simulink model "OCFC"  (R2023a)
settings: Solver=VariableStepAuto  StartTime=0.0  StopTime=200  RelTol=1e-3
libraries: simulink x1, slpidlib x1, SignalEditorBlockLib x1
settings Model: Creator=nineday  LastModifiedBy=nineday
settings ModelReferenceCC: EnableRefExpFcnMdlSchedulingChecks=on

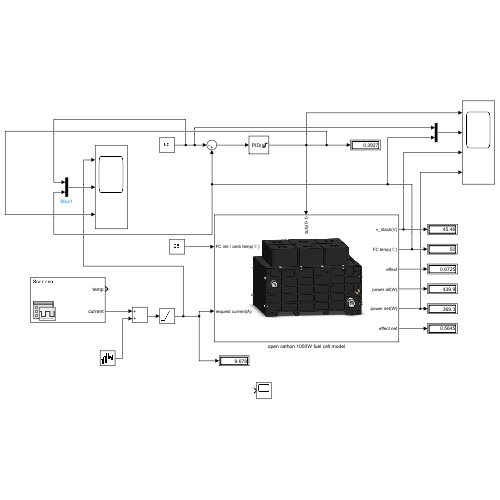
[thumbnail: Simulink's stored preview of the top-level diagram]
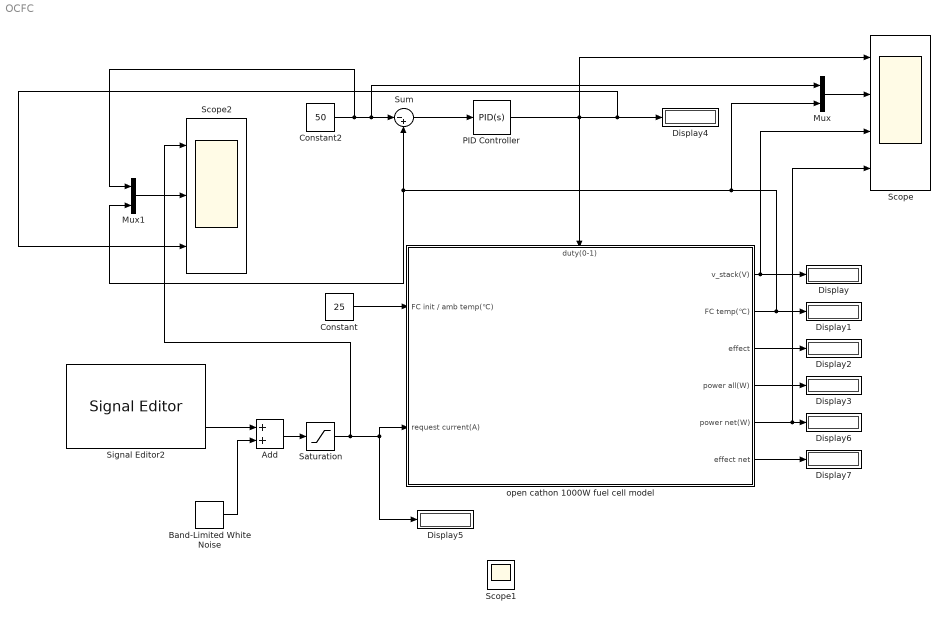
== system OCFC ==
  Add : Sum
  Band-Limited White Noise : simulink/Sources/Band-Limited White Noise  Cov=[0.1]  Ts=0.1  seed=[23341]
  Constant : Constant  Value=25
  Constant2 : Constant  Value=50
  Display{,1..7} (8 alike) : Display
  Mux : Mux  Inputs=2
  Mux1 : Mux  Inputs=2
  PID Controller : slpidlib/PID Controller  Controller=PID  Form=Parallel  TimeDomain=Continuous-time  UseExternalTs=off  SampleTime=-1  IntegratorMethod=Forward Euler  FilterMethod=Forward Euler  ControllerParametersSource=internal  P=1  I=0.1  UseKiTs=off  D=0  N=100  UseFilter=on  TunerSelectOption=Transfer Function Based (PID Tuner App)  InitialConditionSource=internal  InitialConditionForIntegrator=0  InitialConditionForFilter=0  DifferentiatorICPrevScaledInput=0  ExternalReset=none  TrackingMode=off  Kt=1  LimitOutput=on  SatLimitsSource=internal  UpperSaturationLimit=1  LowerSaturationLimit=0  LinearizeAsGain=on  AntiWindupMode=clamping  Kb=1  LimitIntegrator=off  UpperIntegratorSaturationLimit=inf  LowerIntegratorSaturationLimit=-inf  POutMin=[]  POutMax=[]  IOutMin=[]  IOutMax=[]  DOutMin=[]  DOutMax=[]  NOutMin=[]  NOutMax=[]  SumOutMin=[]  SumOutMax=[]  SaturationOutMin=[]  SaturationOutMax=[]  PParamMin=[]  PParamMax=[]  IParamMin=[]  IParamMax=[]  DParamMin=[]  DParamMax=[]  NParamMin=[]  NParamMax=[]  KbParamMin=[]  KbParamMax=[]  KtParamMin=[]  KtParamMax=[]  KbOutMin=[]  KbOutMax=[]  KtOutMin=[]  KtOutMax=[]  IntegratorOutMin=[]  IntegratorOutMax=[]  FilterOutMin=[]  FilterOutMax=[]  SumI1OutMin=[]  SumI1OutMax=[]  SumI2OutMin=[]  SumI2OutMax=[]  SumI3OutMin=[]  SumI3OutMax=[]  SumI4OutMin=[]  SumI4OutMax=[]  SumDOutMin=[]  SumDOutMax=[]  DifferentiatorOutMin=[]  DifferentiatorOutMax=[]  FilterDiffOutCoefMin=[]  FilterDiffOutCoefMax=[]  ReciprocalOutMin=[]  ReciprocalOutMax=[]  SumDenOutMin=[]  SumDenOutMax=[]  SumNumOutMin=[]  SumNumOutMax=[]  DivideOutMin=[]  DivideOutMax=[]  UdiffTsProdOutMin=[]  UdiffTsProdOutMax=[]  NTsProdOutMin=[]  NTsProdOutMax=[]  UintegralTsProdOutMin=[]  UintegralTsProdOutMax=[]  UngainTsProdOutMin=[]  UngainTsProdOutMax=[]  ClampingZeroOutDataTypeStr=Inherit: Inherit via back propagation  ClampingZeroOutMin=[]  ClampingZeroOutMax=[]  FilterDenConstantOutDataTypeStr=Inherit: Inherit via back propagation  FilterDenConstantOutMin=[]  FilterDenConstantOutMax=[]  PCopyOutDataTypeStr=Inherit: Inherit via back propagation  PCopyOutMin=[]  PCopyOutMax=[]  NCopyOutDataTypeStr=Inherit: Inherit via back propagation  NCopyOutMin=[]  NCopyOutMax=[]  IntegratorContinuousStateAttributes=''  IntegratorStateMustResolveToSignalObject=off  IntegratorRTWStateStorageClass=Auto  FilterContinuousStateAttributes=''  FilterStateMustResolveToSignalObject=off  FilterRTWStateStorageClass=Auto  ParallelPVariant=InternalParameters  IdealPVariant=Disabled  IVariant=InternalParameters  DVariant=InternalParameters  IntegratorVariant=Continuous  SatVariant=Enabled  AWVariant=ContClampingParallel  PCopyVariant=Disabled  TRVariant=Disabled  FdbkBlocksVariant=Forward  IdealPFdbkVariant=Disabled  SatFdbkVariant=Disabled  DerivativeFilterVariant=ContFilter  NVariant=InternalParameters  NCopyVariant=Disabled  FilterICVariant=InternalICsFilter  IntegratorICVariant=InternalICs  ExternalResetVariant=Disabled  TRSumVariant=Passthrough  SumFdbkVariant=Disabled  SumVariant=Sum_PID  TsampFilterVariant=InternalTs  TsampNgainVariant=Passthrough  TsampIntegralVariant=Disabled_SignalSpec  ExternalSaturationOutDataTypeStr=Inherit: Same as second input
  Saturation : Saturate  UpperLimit=30  LowerLimit=0
  Scope : Scope  NumInputPorts=4
  Scope1 : Scope
  Scope2 : Scope  NumInputPorts=3
  Signal Editor2 : SignalEditorBlockLib/Signal Editor  FileName=testacurrent.mat  ActiveScenario=Scenario  ActiveSignal=temp  IsBus=off  OutputBusObjectStr=Bus: BusObject  SampleTime=0  Interpolate=off  ZeroCross=off  OutputAfterFinalValue=Setting to zero  Unit=inherit  PreserveSignalName=on  ApplySigPropsToAllScenarios=on
  Sum : Sum  Inputs=|-+
  open cathon 1000W fuel cell model : Subsystem
      settings: PortSchema="{\"entries\":[{\"content\":{\"sides\":[{\"content\":{\"connectorIds\":[\"In1\",\"In2\"]},\"type\":\"ConnectorPlacement.EquallySpacedRectSide\",\"uuid\":\"ba3cf3bf-5a88-4595-bc65-1473d8f13f85\"},{\"content\":{\"connectorIds\":[\"Out1\",\"Out2\",\"Out3\",\"Out4\",\"Out5\",\"Out6\"],\"side\":\"RIGHT\"},\"type\":\"ConnectorPlacement.EquallySpacedRectSide\",\"uuid\":\"62fe74ea-737d-441a-9df1-d302b55047a0\"},{\"content\":{\"connectorIds\":[\"In3\"],\"side\":\"TOP\"},\"type\":\"ConnectorPlacement.EquallySpacedRectSide\",\"uuid\":\"ed0d130b-e41c-4103-82f4-ed869a0f0769\"}]},\"type\":\"ConnectorPlacement.EquallySpacedConnector\",\"uuid\":\"d27583e0-2019-41e5-9706-fbc9de0d1b1c\"}],\"packageUris\":[\"http://schema.mathworks.com/mf0/Connector/R2020b\"],\"version\":\"1.0\"}"
      mask Display: image('$imagefile'); % 使用工具条上的 "编辑图像" 进行更改。
  wires:
  Constant/1 -> open cathon 1000W fuel cell model/1(FC init / amb temp(℃))
  Add/1 -> Saturation/1
  open cathon 1000W fuel cell model/1(v_stack(V)) -> Scope/3, Display/1
  open cathon 1000W fuel cell model/3(effect) -> Display2/1
  open cathon 1000W fuel cell model/4(power all(W)) -> Display3/1
  Sum/1 -> PID Controller/1
  PID Controller/1 -> open cathon 1000W fuel cell model/3(duty(0-1)), Scope/1, Scope2/3, Display4/1
  Constant2/1 -> Mux1/1, Mux/1, Sum/1
  Mux/1 -> Scope/2
  open cathon 1000W fuel cell model/5(power net(W)) -> Scope/4, Display6/1
  open cathon 1000W fuel cell model/6(effect net) -> Display7/1
  Signal Editor2/2 -> Add/1
  Band-Limited White Noise/1 -> Add/2
  Saturation/1 -> Scope2/1, open cathon 1000W fuel cell model/2(request current(A)), Display5/1
  open cathon 1000W fuel cell model/2(FC temp(℃)) -> Mux/2, Sum/2, Mux1/2, Display1/1
  Mux1/1 -> Scope2/2

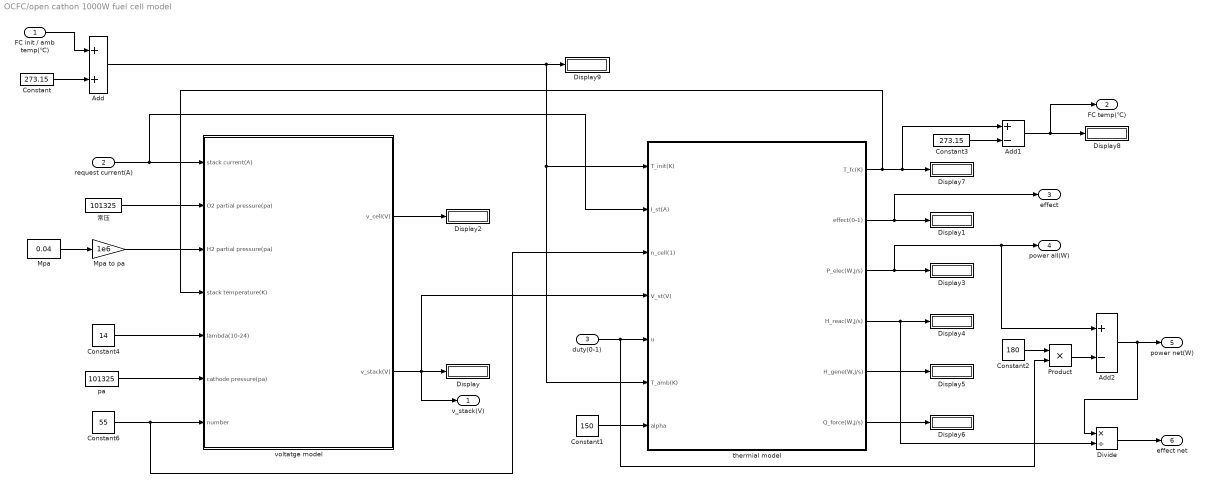
== system OCFC/open cathon 1000W fuel cell model ==
  FC init / amb temp(℃) : Inport
  request current(A) : Inport  Port=2
  duty(0-1) : Inport  Port=3
  Add : Sum
  Add1 : Sum  Inputs=+-
  Add2 : Sum  Inputs=+-
  Constant : Constant  Value=273.15
  Constant1 : Constant  Value=150
  Constant2 : Constant  Value=180
  Constant3 : Constant  Value=273.15
  Constant4 : Constant  Value=14
  Constant6 : Constant  Value=55
  Display{,1..9} (10 alike) : Display
  Divide : Product  Inputs=*/
  Mpa : Constant  Value=0.04
  Mpa to pa : Gain  Gain=1e6
  Product : Product
  pa : Constant  Value=101325
  thermial model : Subsystem
  voltatge model : Subsystem
  常压 : Constant  Value=101325
  v_stack(V) : Outport
  FC temp(℃) : Outport  Port=2
  effect : Outport  Port=3
  power all(W) : Outport  Port=4
  power net(W) : Outport  Port=5
  effect net : Outport  Port=6
  wires:
  Constant6/1 -> thermial model/3(n_cell(1)), voltatge model/7(number)
  Constant/1 -> Add/2
  voltatge model/2(v_stack(V)) -> v_stack(V)/1, Display/1, thermial model/4(V_st(V))
  thermial model/1(T_fc(K)) -> Add1/1, Display7/1, voltatge model/4(stack temperature(K))
  Constant4/1 -> voltatge model/5(lambda(10-24))
  Mpa to pa/1 -> voltatge model/3(H2 partial pressure(pa))
  voltatge model/1(v_cell(V)) -> Display2/1
  常压/1 -> voltatge model/2(O2 partial pressure(pa))
  thermial model/3(P_elec(W,J/s)) -> Add2/1, power all(W)/1, Display3/1
  request current(A)/1 -> voltatge model/1(stack current(A)), thermial model/2(I_st(A))
  Mpa/1 -> Mpa to pa/1
  pa/1 -> voltatge model/6(cathode pressure(pa))
  Constant3/1 -> Add1/2
  Add/1 -> thermial model/6(T_amb(K)), thermial model/1(T_init(K)), Display9/1
  thermial model/5(H_gene(W,J/s)) -> Display5/1
  thermial model/2(effect(0-1)) -> effect/1, Display1/1
  thermial model/4(H_reac(W,J/s)) -> Divide/2, Display4/1
  thermial model/6(Q_force(W,J/s)) -> Display6/1
  Constant1/1 -> thermial model/7(alpha)
  FC init / amb temp(℃)/1 -> Add/1
  Add1/1 -> FC temp(℃)/1, Display8/1
  duty(0-1)/1 -> Product/2, thermial model/5(u)
  Add2/1 -> Divide/1, power net(W)/1
  Product/1 -> Add2/2
  Constant2/1 -> Product/1
  Divide/1 -> effect net/1

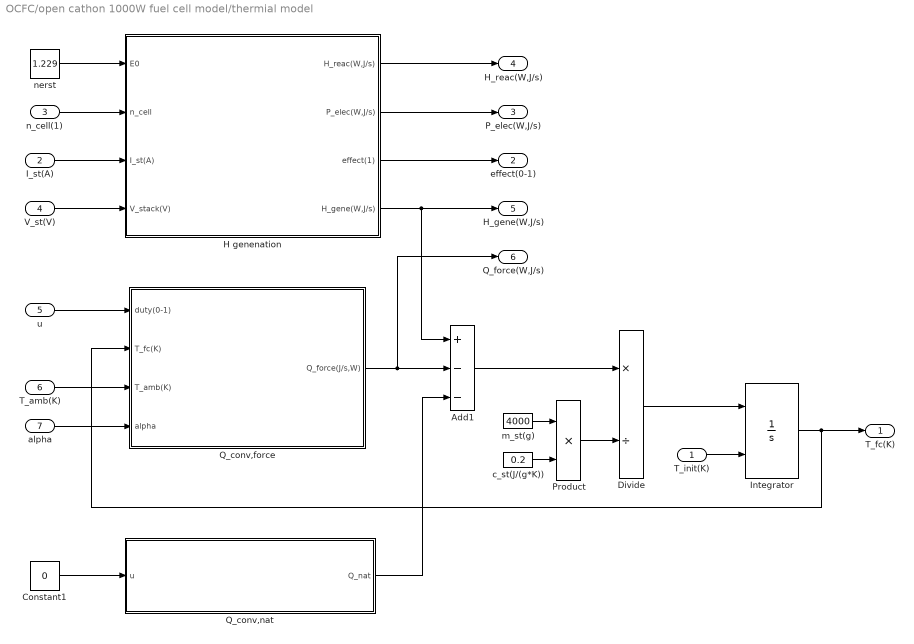
== system OCFC/open cathon 1000W fuel cell model/thermial model ==
  T_init(K) : Inport
  I_st(A) : Inport  Port=2
  n_cell(1) : Inport  Port=3
  V_st(V) : Inport  Port=4
  u : Inport  Port=5
  T_amb(K) : Inport  Port=6
  alpha : Inport  Port=7
  Add1 : Sum  Inputs=+--
  Constant1 : Constant  Value=0
  Divide : Product  Inputs=*/
  H genenation : Subsystem
  Integrator : Integrator  InitialConditionSource=external  LimitOutput=on  UpperSaturationLimit=373.15  LowerSaturationLimit=273.15
  Product : Product
  Q_conv,force : Subsystem
  Q_conv,nat : MATLAB Function  TreatAsAtomicUnit=on
  c_st(J/(g*K)) : Constant  Value=0.2
  m_st(g) : Constant  Value=4000
  nerst : Constant  Value=1.229
  T_fc(K) : Outport
  effect(0-1) : Outport  Port=2
  P_elec(W,J/s) : Outport  Port=3
  H_reac(W,J/s) : Outport  Port=4
  H_gene(W,J/s) : Outport  Port=5
  Q_force(W,J/s) : Outport  Port=6
  wires:
  c_st(J/(g*K))/1 -> Product/2
  n_cell(1)/1 -> H genenation/2(n_cell)
  Q_conv,force/1(Q_force(J/s,W)) -> Q_force(W,J/s)/1, Add1/2
  Product/1 -> Divide/2
  nerst/1 -> H genenation/1(E0)
  m_st(g)/1 -> Product/1
  Q_conv,nat/1(Q_nat) -> Add1/3
  Constant1/1 -> Q_conv,nat/1(u)
  H genenation/3(effect(1)) -> effect(0-1)/1
  T_init(K)/1 -> Integrator/2
  Divide/1 -> Integrator/1
  H genenation/4(H_gene(W,J/s)) -> H_gene(W,J/s)/1, Add1/1
  Add1/1 -> Divide/1
  I_st(A)/1 -> H genenation/3(I_st(A))
  T_amb(K)/1 -> Q_conv,force/3(T_amb(K))
  Integrator/1 -> T_fc(K)/1, Q_conv,force/2(T_fc(K))
  u/1 -> Q_conv,force/1(duty(0-1))
  H genenation/1(H_reac(W,J/s)) -> H_reac(W,J/s)/1
  V_st(V)/1 -> H genenation/4(V_stack(V))
  H genenation/2(P_elec(W,J/s)) -> P_elec(W,J/s)/1
  alpha/1 -> Q_conv,force/4(alpha)

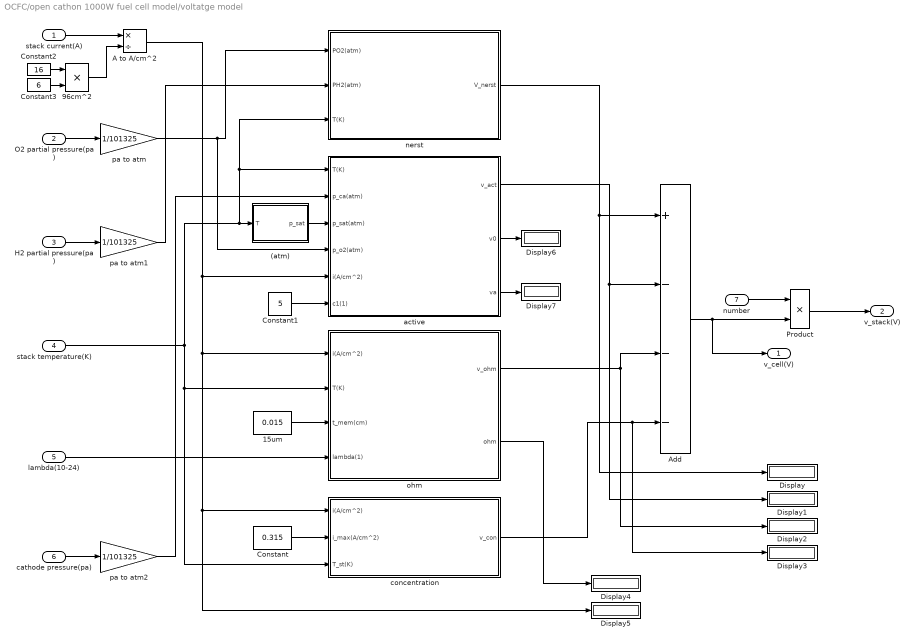
== system OCFC/open cathon 1000W fuel cell model/voltatge model ==
  stack current(A) : Inport
  O2 partial pressure(pa) : Inport  Port=2
  H2 partial pressure(pa) : Inport  Port=3
  stack temperature(K) : Inport  Port=4
  lambda(10-24) : Inport  Port=5
  cathode pressure(pa) : Inport  Port=6
  number : Inport  Port=7
  (atm) : MATLAB Function  TreatAsAtomicUnit=on
  15um : Constant  Value=0.015
  96cm^2 : Product
  A to A/cm^2 : Product  Inputs=*/
  Add : Sum  Inputs=+---
  Constant : Constant  Value=0.315
  Constant1 : Constant  Value=5
  Constant2 : Constant  Value=16
  Constant3 : Constant  Value=6
  Display{,1..7} (8 alike) : Display
  Product : Product
  active : Subsystem
  concentration : Subsystem
  nerst : Subsystem
  ohm : Subsystem
  pa to atm : Gain  Gain=1/101325
  pa to atm1 : Gain  Gain=1/101325
  pa to atm2 : Gain  Gain=1/101325
  v_cell(V) : Outport
  v_stack(V) : Outport  Port=2
  wires:
  Add/1 -> v_cell(V)/1, Product/2
  stack temperature(K)/1 -> active/1(T(K)), nerst/3(T(K)), (atm)/1(T), concentration/3(T_st(K)), ohm/2(T(K))
  pa to atm2/1 -> active/2(p_ca(atm))
  concentration/1(v_con) -> Display3/1, Add/4
  ohm/1(v_ohm) -> Add/3, Display2/1
  H2 partial pressure(pa)/1 -> pa to atm1/1
  (atm)/1(p_sat) -> active/3(p_sat(atm))
  pa to atm/1 -> nerst/1(PO2(atm)), active/4(p_o2(atm))
  pa to atm1/1 -> nerst/2(PH2(atm))
  number/1 -> Product/1
  O2 partial pressure(pa)/1 -> pa to atm/1
  Constant/1 -> concentration/2(i_max(A/cm^2))
  lambda(10-24)/1 -> ohm/4(lambda(1))
  stack current(A)/1 -> A to A/cm^2/1
  Product/1 -> v_stack(V)/1
  cathode pressure(pa)/1 -> pa to atm2/1
  15um/1 -> ohm/3(t_mem(cm))
  active/1(v_act) -> Display1/1, Add/2
  Constant2/1 -> 96cm^2/1
  Constant3/1 -> 96cm^2/2
  96cm^2/1 -> A to A/cm^2/2
  nerst/1(V_nerst) -> Display/1, Add/1
  ohm/2(ohm) -> Display4/1
  A to A/cm^2/1 -> Display5/1, concentration/1(i(A/cm^2)), ohm/1(i(A/cm^2)), active/5(i(A/cm^2))
  Constant1/1 -> active/6(c1(1))
  active/2(v0) -> Display6/1
  active/3(va) -> Display7/1

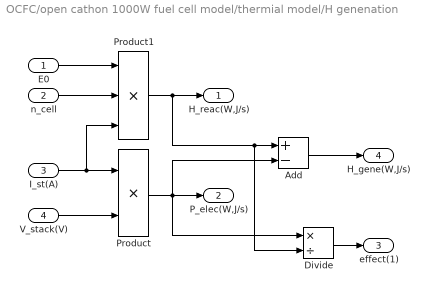
== system OCFC/open cathon 1000W fuel cell model/thermial model/H genenation ==
  E0 : Inport
  n_cell : Inport  Port=2
  I_st(A) : Inport  Port=3
  V_stack(V) : Inport  Port=4
  Add : Sum  Inputs=+-
  Divide : Product  Inputs=*/
  Product : Product
  Product1 : Product  Inputs=3
  H_reac(W,J/s) : Outport
  P_elec(W,J/s) : Outport  Port=2
  effect(1) : Outport  Port=3
  H_gene(W,J/s) : Outport  Port=4
  wires:
  V_stack(V)/1 -> Product/2
  I_st(A)/1 -> Product1/3, Product/1
  n_cell/1 -> Product1/2
  E0/1 -> Product1/1
  Product1/1 -> Divide/2, Add/1, H_reac(W,J/s)/1
  Product/1 -> Divide/1, Add/2, P_elec(W,J/s)/1
  Add/1 -> H_gene(W,J/s)/1
  Divide/1 -> effect(1)/1

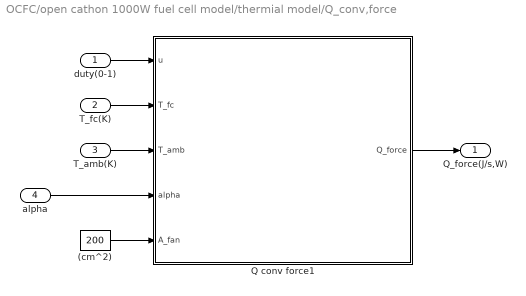
== system OCFC/open cathon 1000W fuel cell model/thermial model/Q_conv,force ==
  duty(0-1) : Inport
  T_fc(K) : Inport  Port=2
  T_amb(K) : Inport  Port=3
  alpha : Inport  Port=4
  (cm^2) : Constant  Value=200
  Q conv force1 : MATLAB Function  TreatAsAtomicUnit=on
  Q_force(J/s,W) : Outport
  wires:
  T_fc(K)/1 -> Q conv force1/2(T_fc)
  T_amb(K)/1 -> Q conv force1/3(T_amb)
  Q conv force1/1(Q_force) -> Q_force(J/s,W)/1
  duty(0-1)/1 -> Q conv force1/1(u)
  alpha/1 -> Q conv force1/4(alpha)
  (cm^2)/1 -> Q conv force1/5(A_fan)

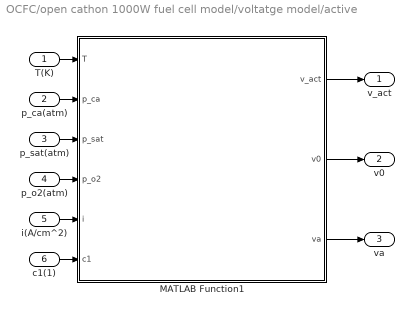
== system OCFC/open cathon 1000W fuel cell model/voltatge model/active ==
  T(K) : Inport
  p_ca(atm) : Inport  Port=2
  p_sat(atm) : Inport  Port=3
  p_o2(atm) : Inport  Port=4
  i(A/cm^2) : Inport  Port=5
  c1(1) : Inport  Port=6
  MATLAB Function1 : MATLAB Function  TreatAsAtomicUnit=on
  v_act : Outport
  v0 : Outport  Port=2
  va : Outport  Port=3
  wires:
  i(A/cm^2)/1 -> MATLAB Function1/5(i)
  p_ca(atm)/1 -> MATLAB Function1/2(p_ca)
  p_sat(atm)/1 -> MATLAB Function1/3(p_sat)
  T(K)/1 -> MATLAB Function1/1(T)
  p_o2(atm)/1 -> MATLAB Function1/4(p_o2)
  MATLAB Function1/1(v_act) -> v_act/1
  c1(1)/1 -> MATLAB Function1/6(c1)
  MATLAB Function1/2(v0) -> v0/1
  MATLAB Function1/3(va) -> va/1

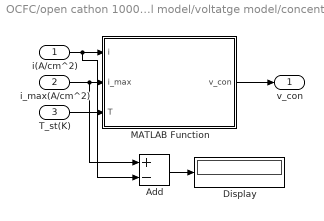
== system OCFC/open cathon 1000W fuel cell model/voltatge model/concentration ==
  i(A/cm^2) : Inport
  i_max(A/cm^2) : Inport  Port=2
  T_st(K) : Inport  Port=3
  Add : Sum  Inputs=+-
  Display : Display
  MATLAB Function : MATLAB Function  TreatAsAtomicUnit=on
  v_con : Outport
  wires:
  i_max(A/cm^2)/1 -> Add/1, MATLAB Function/2(i_max)
  i(A/cm^2)/1 -> Add/2, MATLAB Function/1(i)
  MATLAB Function/1(v_con) -> v_con/1
  T_st(K)/1 -> MATLAB Function/3(T)
  Add/1 -> Display/1

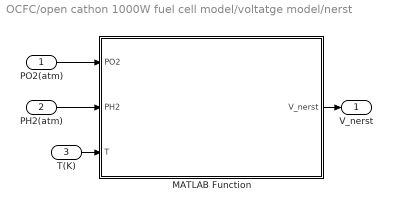
== system OCFC/open cathon 1000W fuel cell model/voltatge model/nerst ==
  PO2(atm) : Inport
  PH2(atm) : Inport  Port=2
  T(K) : Inport  Port=3
  MATLAB Function : MATLAB Function  TreatAsAtomicUnit=on
  V_nerst : Outport
  wires:
  PO2(atm)/1 -> MATLAB Function/1(PO2)
  T(K)/1 -> MATLAB Function/3(T)
  MATLAB Function/1(V_nerst) -> V_nerst/1
  PH2(atm)/1 -> MATLAB Function/2(PH2)

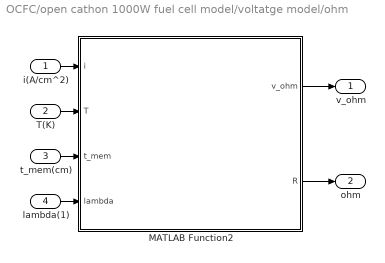
== system OCFC/open cathon 1000W fuel cell model/voltatge model/ohm ==
  i(A/cm^2) : Inport
  T(K) : Inport  Port=2
  t_mem(cm) : Inport  Port=3
  lambda(1) : Inport  Port=4
  MATLAB Function2 : MATLAB Function  TreatAsAtomicUnit=on
  v_ohm : Outport
  ohm : Outport  Port=2
  wires:
  t_mem(cm)/1 -> MATLAB Function2/3(t_mem)
  MATLAB Function2/1(v_ohm) -> v_ohm/1
  T(K)/1 -> MATLAB Function2/2(T)
  lambda(1)/1 -> MATLAB Function2/4(lambda)
  i(A/cm^2)/1 -> MATLAB Function2/1(i)
  MATLAB Function2/2(R) -> ohm/1

== matlab function OCFC/open cathon 1000W fuel cell model/voltatge model/active/MATLAB Function1 ==
  data: T input; v_act output; p_ca input; p_sat input; p_o2 input; i input; c1 input; v0 output; va output
function [v_act,v0,va] = active(T,p_ca,p_sat,p_o2,i,c1)

v0 = 0.279-8.5e-4*(T-298.15)+4.308e-5*T*(log((p_ca-p_sat)/1.01325)+0.5*log(0.1173*(p_ca-p_sat)/1.01325));

va = (-1.618e-5*T + 1.618e-2)*(p_o2/0.1173+p_sat)^2 + (1.8e-4*T-0.166)*(p_o2/0.1173+p_sat) + (-5.8e-4*T+0.5736);

v_act = v0 + va*(1-exp(-c1*i));

== matlab function OCFC/open cathon 1000W fuel cell model/voltatge model/nerst/MATLAB Function ==
  data: PO2 input; PH2 input; T input; V_nerst output
function V_nerst = nerst(PO2,PH2,T )

V_nerst = 1.229-8.5*10^(-4)*(T-298.15)+4.3085*10^(-5)*T*(log(PH2)+0.5*log(PO2));

== matlab function OCFC/open cathon 1000W fuel cell model/voltatge model/(atm) ==
  data: T input; p_sat output
function p_sat = saturation(T)
p_sat = exp(23.196-3816.44/(T-46.13))/101325;

== matlab function OCFC/open cathon 1000W fuel cell model/voltatge model/ohm/MATLAB Function2 ==
  data: i input; T input; v_ohm output; t_mem input; lambda input; R output
function [v_ohm,R] = ohm(i, T , t_mem, lambda)

sigma_m = (0.514*lambda - 0.033)*exp(1268*(1/303-1/T));

R_m = t_mem/sigma_m;

R_c = 0;

%R = R_m+R_c;

R=0.15; %R/cm^2 典型值
v_ohm = i*R;

== matlab function OCFC/open cathon 1000W fuel cell model/voltatge model/concentration/MATLAB Function ==
  data: i input; v_con output; i_max input; T input
function v_con = concentration(i,i_max,T)
R=8.314;    %J/(mol·K)  气体常数
F=96485;    %C/mol, A*s/mol 法拉第常数
B=R*T/(2*F);
v_con = B*log(i_max/(i_max-i));

== matlab function OCFC/open cathon 1000W fuel cell model/thermial model/Q_conv,nat ==
  data: u input; Q_nat output
function Q_nat = conv_nat(u)

Q_nat = u;

== matlab function OCFC/open cathon 1000W fuel cell model/thermial model/Q_conv,force/Q conv force1 ==
  data: u input; Q_force output; T_fc input; T_amb input; alpha input; A_fan input
function Q_force = conv_force(u,T_fc, T_amb, alpha, A_fan)

rho_air = 1.29e-3;  % 空气密度   g/cm^3
C_air = 1.004;      % 空气比热容 J/(g*K)

% u         占空比 0-1
% T_fc      电堆温度 K
% T_amb     环境温度 K
% alpha     经验系数 1
% A_fan     有效换热面积 cm^2


Q_force = alpha*u*rho_air*C_air*A_fan*(T_fc-T_amb);
